simulink model "VehicleFollowing"  (R2020a)
settings: Solver=VariableStepAuto  StartTime=0.0  StopTime=30  RelTol=1e-3
InitFcn:
  | load("bus.mat");
model workspace (MAT data in the model file):
  Acc_command = Simulink.Parameter
  Acc_command.DataType = 'auto'
  Acc_command.Dimensions = [0 0]
  AngIn_command = Simulink.Parameter
  AngIn_command.DataType = 'auto'
  AngIn_command.Dimensions = [0 0]
  Dece_command = Simulink.Parameter
  Dece_command.DataType = 'auto'
  Dece_command.Dimensions = [0 0]
libraries: autolibutils x4, autolibshared x3, simulink x3, drivinglib x2, drivingscenarioandsensors x2, vrlib x2, vehdynlibsteering x1, mpcadaslib x1, robotalgslib x1
(part 1 of 3)
settings Model: PacingRate=1.100000  OrderedModelArguments=off  Creator=shiqihang  LastModifiedBy=shiqihang
settings SolverCC: AlgebraicLoopSolver=LineSearch
settings DebuggingCC: AlgebraicLoopMsg=none

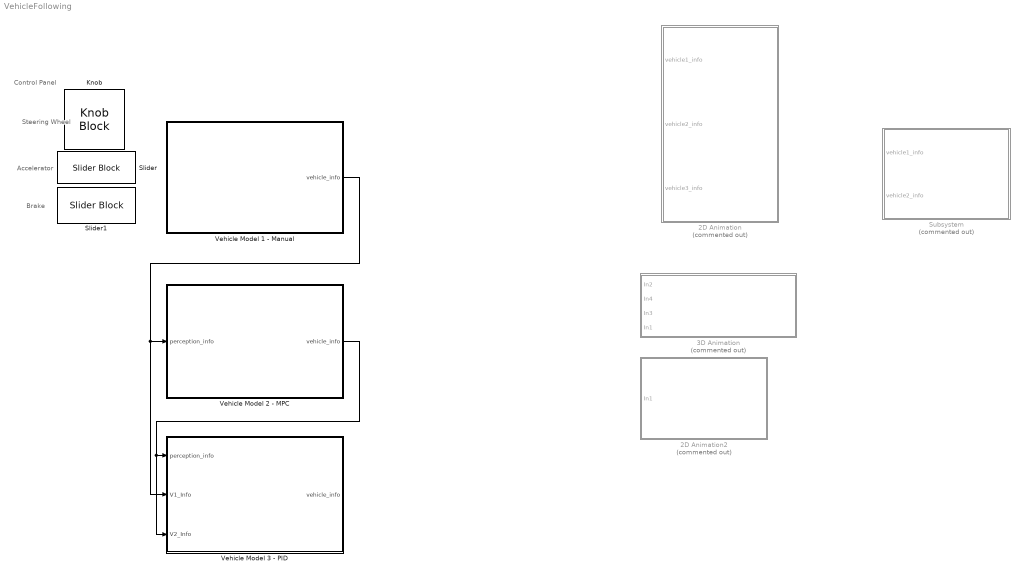
== system VehicleFollowing ==
  note: Steering
      | Wheel
  note: Control Panel
  note: Accelerator
  note: Brake
  2D Animation : Subsystem  Commented=on  TreatAsAtomicUnit=on  SystemSampleTime=0.02
  2D Animation2 : Subsystem  Commented=on
  3D Animation : Subsystem  Commented=on
  Knob : KnobBlock  ScaleMin=-2  ScaleMax=2
  Slider : SliderBlock
  Slider1 : SliderBlock
  Subsystem : Subsystem  Commented=on
  Vehicle Model 1 - Manual : Subsystem  mask{X_init=150, xdot_init=10, Y_init=-2.5, ydot_init=0, AngIn_command=-0.006511027018229143, Acc_command=0.3429878048780488, Dece_command=0}
      mask prompts: X_init "Initial X Position"; xdot_init "Initial Longitudinal Velocity"; Y_init "Initial Y Position"; ydot_init "Initial Lateral Velocity"; AngIn_command "Angle Command"; Acc_command "Acc Command"; Dece_command "Dece Command"
      mask Display: image('$imagefile'); % Use "Edit Image" on toolstrip to change.
  Vehicle Model 2 - MPC : Subsystem  mask{X_init=40, xdot_init=5, Y_init=-2.5, ydot_init=0}
      mask prompts: X_init "Initial X Position"; xdot_init "Initial Longitudinal Velocity"; Y_init "Initial Y Position"; ydot_init "Initial Lateral Velocity"
      mask TypeOptions X_init: Initial Position Z/Value
      mask TypeOptions xdot_init: Initial Speed/Value
      mask Display: image('$imagefile'); % Use "Edit Image" on toolstrip to change.
  Vehicle Model 3 - PID : Subsystem  mask{X_init=0, xdot_init=20, Y_init=-2.5, ydot_init=0}
      mask prompts: X_init "Initial X Position"; xdot_init "Initial Longitudinal Velocity"; Y_init "Initial Y Position"; ydot_init "Initial Lateral Velocity"
      mask TypeOptions X_init: Initial Position Z/Value
      mask TypeOptions xdot_init: Initial Speed/Value
      mask Display: image('C:\Users\qihan\Desktop\Git\Vehicle-following-model-with-3DAnimation\resources\image\vehicle.png'); % Use "Edit Image" on toolstrip to change.
  wires:
  Vehicle Model 1 - Manual/1(vehicle_info) -> Vehicle Model 2 - MPC/1(perception_info), Vehicle Model 3 - PID/2(V1_Info)
  Vehicle Model 2 - MPC/1(vehicle_info) -> Vehicle Model 3 - PID/3(V2_Info), Vehicle Model 3 - PID/1(perception_info)

== system VehicleFollowing/2D Animation ==
  vehicle1_info : Inport
  vehicle2_info : Inport  Port=2
  vehicle3_info : Inport  Port=3
  Bus Selector : BusSelector  OutputSignals=InertFrm.Cg.Disp.X,InertFrm.Cg.Disp.Y,InertFrm.Cg.Ang.psi  OutputAsBus=on
  Bus Selector1 : BusSelector  OutputSignals=X,Y,psi  OutputAsBus=on
  Bus Selector2 : BusSelector  OutputSignals=InertFrm.Cg.Disp.X,InertFrm.Cg.Disp.Y,InertFrm.Cg.Ang.psi  OutputAsBus=on
  MATLAB Function : MATLAB Function  TreatAsAtomicUnit=on
      mask init:
      | close all;
      | figure('units','normalized','outerposition',[0 0 1 1]);
      | grid on
      | axis equal
      | hold on
  wires:
  Bus Selector/1 -> MATLAB Function/1(V1_Pose)
  vehicle1_info/1 -> Bus Selector/1
  vehicle2_info/1 -> Bus Selector1/1
  Bus Selector1/1 -> MATLAB Function/2(V2_Pose)
  vehicle3_info/1 -> Bus Selector2/1
  Bus Selector2/1 -> MATLAB Function/3(V3_Pose)

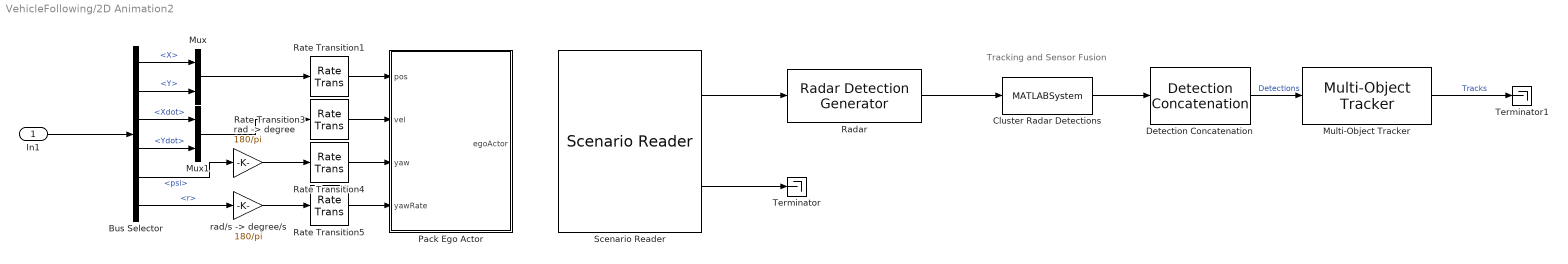
== system VehicleFollowing/2D Animation2 ==
  note: Tracking and Sensor Fusion
  In1 : Inport
  Bus Selector : BusSelector  OutputSignals=InertFrm.Cg.Disp.X,InertFrm.Cg.Disp.Y,InertFrm.Cg.Vel.Xdot,InertFrm.Cg.Vel.Ydot,InertFrm.Cg.Ang.psi,BdyFrm.Cg.AngVel.r
  Cluster Radar Detections : MATLABSystem  System=helperClusterDetections  ClusterSize=5  BusNameSource=Auto  BusName=BusClusterDetections  SimulateUsing=Interpreted execution
      mask Type: helperClusterDetections
      mask Display:
      | disp(['Detection' char(10) 'Clustering']);
      | port_label('input',1,'In');
      | port_label('output',1,'Out');
  Detection Concatenation : drivinglib/Detection Concatenation  NumInputs=1  BusNameSource=Auto  BusName=BusDetectionConcatenation1  SimulateUsing=Interpreted execution
      settings: SourceProductBaseCode=DR
  Multi-Object Tracker : drivinglib/Multi-Object Tracker  TrackerIndex=uint32( 0 )  FilterInitializationFcn=helperInitSimulinkDemoFilter  AssignmentThreshold=50  ConfirmationThreshold=[ 2, 3 ]  DeletionThreshold=[5,5]  MaxNumTracks=20  MaxNumSensors=8  StateParams=struct  TimeInputSource=Auto  HasCostMatrixInput=off  HasDetectableTrackIDsInput=off  BusNameSource=Auto  BusName=BusMultiObjectTracker1  TentativeTracksOutputPort=off  AllTracksOutputPort=off  SimulateUsing=Interpreted execution
      settings: SourceProductBaseCode=DR
  Mux : Mux  Inputs=2
  Mux1 : Mux  Inputs=2
  Pack Ego Actor : MATLAB Function  TreatAsAtomicUnit=on
  Radar : drivingscenarioandsensors/Radar Detection Generator  SensorIndex=1  UpdateInterval=0.1  SensorLocation=[3.7 0]  Height=0.2  Yaw=0  Pitch=0  Roll=0  BusNameSource=Auto  BusName=BusRadarDetectionGenerator  MaxNumDetectionsSource=Property  MaxNumDetections=50  DetectionCoordinates=Ego Cartesian  SimulateUsing=Interpreted execution  AzimuthResolution=4  ElevationResolution=10  RangeResolution=2.5  RangeRateResolution=0.5  AzimuthBiasFraction=0.1  ElevationBiasFraction=0.1  RangeBiasFraction=0.05  RangeRateBiasFraction=0.05  FieldOfView=[20 5]  MaxRange=100  RangeRateLimits=[-100 100]  DetectionProbability=0.9  FalseAlarmRate=1e-06  ReferenceRange=100  ReferenceRCS=0  HasElevation=off  HasRangeRate=on  HasNoise=on  HasFalseAlarms=on  HasOcclusion=on  InitialSeedSource=Repeatable  InitialSeed=0  UsedSeed=0  ActorProfilesSource=MATLAB expression  ActorProfilesParameters=driving.internal.ActorProfilesRadarParameters  ActorProfilesExpression=[struct('ActorID',1,'ClassID',1,'Length',4.7,'Width',1.8,'Height',1.4,'OriginOffset',[-1.35 0 0],'MeshVertices',[3.7 -0.9 1.4;3.7 0.9 1.4;-1 0.9 1.4;-1 -0.9 1.4;3.7 -0.9 0;3.7 0.9 0;-1 0.9 0;-1 -0.9 0],'MeshFaces',[6 2 1;1 5 6;8 4 3;3 7 8;6 7 3;3 2 6;5 1 4;4 8 5;4 1 2;2 3 4;7 6 5;5 8 7],'RCSPattern',[10 10;10 10],'RCSAzimuthAngles',[-180 180],'RCSElevationAngles',[-90 90]); struct('ActorID',2,'ClassID',1,'Length',4.7,'Width',1.8,'Height',1.4,'OriginOffset',[-1.35 0 0],'MeshVertices',[3.7 -0.9 1.4;3.7 0.9 1.4;-1 0.9 1.4;-1 -0.9 1.4;3.7 -0.9 0;3.7 0.9 0;-1 0.9 0;-1 -0.9 0],'MeshFaces',[6 2 1;1 5 6;8 4 3;3 7 8;6 7 3;3 2 6;5 1 4;4 8 5;4 1 2;2 3 4;7 6 5;5 8 7],'RCSPattern',[10 10;10 10],'RCSAzimuthAngles',[-180 180],'RCSElevationAngles',[-90 90]); struct('ActorID',3,'ClassID',1,'Length',4.7,'Width',1.8,'Height',1.4,'OriginOffset',[-1.35 0 0],'MeshVertices',[3.7 -0.9 1.4;3.7 0.9 1.4;-1 0.9 1.4;-1 -0.9 1.4;3.7 -0.9 0;3.7 0.9 0;-1 0.9 0;-1 -0.9 0],'MeshFaces',[6 2 1;1 5 6;8 4 3;3 7 8;6 7 3;3 2 6;5 1 4;4 8 5;4 1 2;2 3 4;7 6 5;5 8 7],'RCSPattern',[10 10;10 10],'RCSAzimuthAngles',[-180 180],'RCSElevationAngles',[-90 90])]
      settings: SourceProductBaseCode=DR
  Rate Transition{1,3..5} (4 alike) : RateTransition  OutPortSampleTime=0.1
  Scenario Reader : drivingscenarioandsensors/Scenario Reader  ScenarioSource=From workspace  ScenarioFileName=C:\Users\qihan\Desktop\Git\Vehicle-following-model-with-3DAnimation\roads.mat  ScenarioVariableName=ans  OutputCoordinateSystem=Vehicle coordinates  EgoVehicleSource=Scenario  OrientVehiclesOnRoad=off  EgoVehicleActorID=1  OutputEgoVehiclePose=off  SampleTime=0.1  LaneBoundaryOutput=Ego vehicle lane boundaries  LaneBoundaryDistance=0:0.5:9.5  LaneBoundaryLocation=Center of lane markings  BusNameSource=Auto  BusName=BusActors  BusName2Source=Auto  BusName2=BusVision1  BusName3Source=Auto  BusName3=BusEgoActor  ShowCoordinateLabels=on  SimulateUsing=Interpreted execution
  Terminator : Terminator
  Terminator1 : Terminator
  "rad -> degree" : Gain  Gain=180/pi
  "rad/s -> degree/s" : Gain  Gain=180/pi
  wires:
  Rate Transition1/1 -> Pack Ego Actor/1(pos)
  Mux/1 -> Rate Transition1/1
  Multi-Object Tracker/1 -> Terminator1/1  "Tracks"
  "rad -> degree"/1 -> Rate Transition4/1
  Bus Selector/1 -> Mux/1  "<X>"
  Rate Transition5/1 -> Pack Ego Actor/4(yawRate)
  Mux1/1 -> Rate Transition3/1
  "rad/s -> degree/s"/1 -> Rate Transition5/1
  Bus Selector/5 -> "rad -> degree"/1  "<psi>"
  Bus Selector/4 -> Mux1/2  "<Ydot>"
  Scenario Reader/1 -> Radar/1
  Bus Selector/3 -> Mux1/1  "<Xdot>"
  Bus Selector/2 -> Mux/2  "<Y>"
  Rate Transition3/1 -> Pack Ego Actor/2(vel)
  Bus Selector/6 -> "rad/s -> degree/s"/1  "<r>"
  Detection Concatenation/1 -> Multi-Object Tracker/1  "Detections"
  Scenario Reader/2 -> Terminator/1
  Radar/1 -> Cluster Radar Detections/1
  Cluster Radar Detections/1 -> Detection Concatenation/1
  Rate Transition4/1 -> Pack Ego Actor/3(yaw)
  In1/1 -> Bus Selector/1

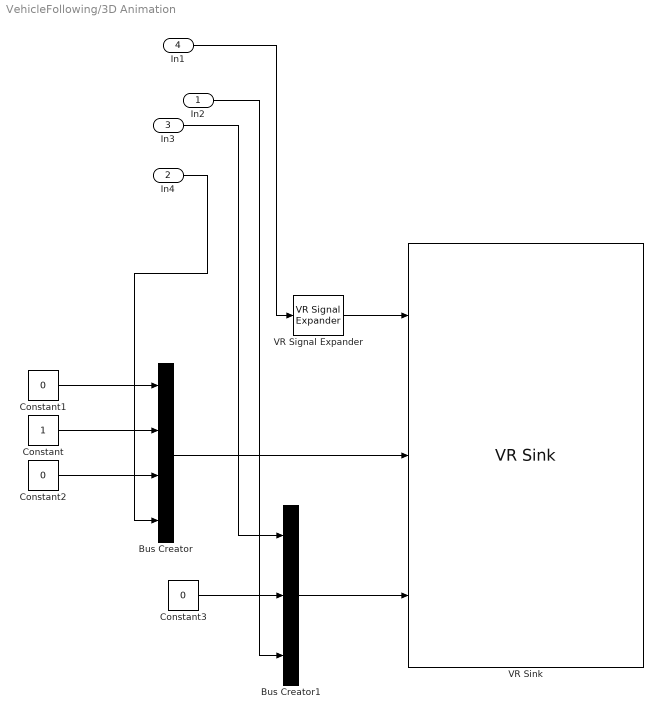
== system VehicleFollowing/3D Animation ==
  In2 : Inport
  In4 : Inport  Port=2
  In3 : Inport  Port=3
  In1 : Inport  Port=4
  Bus Creator : BusCreator  Inputs=4
  Bus Creator1 : BusCreator  Inputs=3
  Constant : Constant
  Constant1 : Constant  Value=0
  Constant2 : Constant  Value=0
  Constant3 : Constant  Value=0
  VR Signal Expander : vrlib/VR Signal Expander  outwidth=3  outidx=[3]
  VR Sink : vrlib/VR Sink  InstantiateOnLoad=on  SampleTime=0.02  ViewEnable=on  RemoteChange=off  RemoteView=off  FieldsWritten=Car_Red.translation.3.1.1.double#Car_Blue.rotation.4.1.1.double#Car_Blue.translation.3.1.1.double  WorldFileName=PlatoonWorld.WRL  AutoView=off  VideoDimensions=[]  AllowVariableSize=off
  wires:
  Constant/1 -> Bus Creator/2
  Constant1/1 -> Bus Creator/1
  Bus Creator1/1 -> VR Sink/3
  In2/1 -> Bus Creator1/3
  Bus Creator/1 -> VR Sink/2
  In4/1 -> Bus Creator/4
  In1/1 -> VR Signal Expander/1
  Constant3/1 -> Bus Creator1/2
  Constant2/1 -> Bus Creator/3
  VR Signal Expander/1 -> VR Sink/1
  In3/1 -> Bus Creator1/1

== system VehicleFollowing/Subsystem ==
  vehicle1_info : Inport
  vehicle2_info : Inport  Port=2
  Bus Selector : BusSelector  OutputSignals=InertFrm.Cg.Disp.X,InertFrm.Cg.Disp.Y,InertFrm.Cg.Ang.psi  OutputAsBus=on
  Bus Selector1 : BusSelector  OutputSignals=X,Y,psi  OutputAsBus=on
  Collision Detection : MATLABSystem  System=collision_detection  v1_frame=[ 4, 2 ]  v2_frame=[ 4, 2 ]  SimulateUsing=Interpreted execution
      mask Type: collision_detection
      mask Display:
      | disp('collision_detection');
      | port_label('input',1,'v1_pos');
      | port_label('input',2,'v2_pos');
      | port_label('output',1,'collision_flag');
  Stop Simulation : Stop
  wires:
  Collision Detection/1 -> Stop Simulation/1
  vehicle1_info/1 -> Bus Selector/1
  Bus Selector1/1 -> Collision Detection/2
  Bus Selector/1 -> Collision Detection/1
  vehicle2_info/1 -> Bus Selector1/1

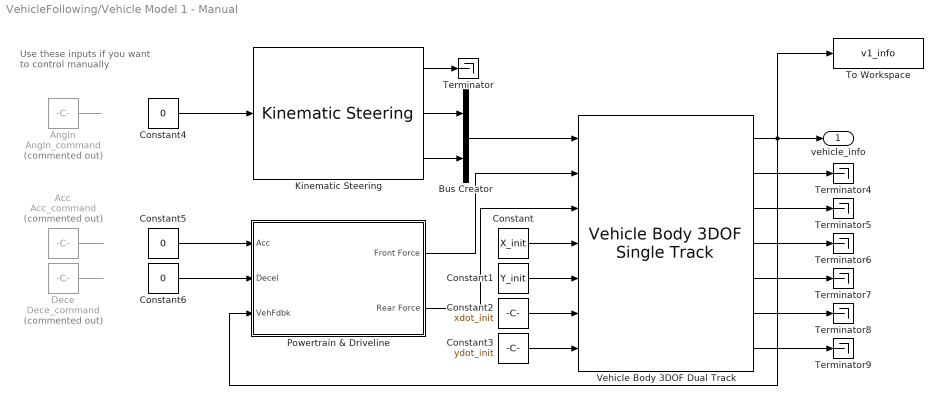
== system VehicleFollowing/Vehicle Model 1 - Manual ==
  note: Use these inputs if
      | you want to control
      | manually
  Acc : Constant  Commented=on  Value=Acc_command
  AngIn : Constant  Commented=on  Value=AngIn_command
  Bus Creator : BusCreator  Inputs=2
  Constant : Constant  Value=X_init
  Constant1 : Constant  Value=Y_init
  Constant2 : Constant  Value=xdot_init
  Constant3 : Constant  Value=ydot_init
  Constant4 : Constant  Value=0
  Constant5 : Constant  Value=0
  Constant6 : Constant  Value=0
  Dece : Constant  Commented=on  Value=Dece_command
  Kinematic Steering : vehdynlibsteering/Kinematic Steering  StrgType=Rack and pinion  StrgRatioType=Constant  Loc=Front  NrmlFctr=0.01  TrckWdth=1  WhlBase=1.524  Db=0  StrgRng=1.25*pi  StrgAngBpts="[-6.2832   -5.0265   -3.7699   -2.5133   -1.2566         0    1.2566    2.5133    3.7699    5.0265    6.2832]"  StrgRatioTbl=|  StrgRatio=100  StrgArmLngth=0.1  RckCsLngth=0.5  TieRodLngth=0.248  D=0.2  PnnRadius=0.0057  PnnRadiusTbl="[0.0055    0.0055    0.0056    0.0057    0.0058    0.0057    0.0057    0.0057    0.0056    0.0055    0.0055]"  RodLngth=0.1  ParaArmLngth=0.9  aMode=2
      | [13.5000   13.3750   13.2500   13.1250   13.0000   13.0000   13.0000   13.1250   13.2500   13.3750   13.5000
      | ]
  Powertrain & Driveline : Subsystem
      mask Display: image('vdbslibpt.png');
  Terminator{,4..9} (7 alike) : Terminator
  To Workspace : ToWorkspace  VariableName=v1_info  SaveFormat=Timeseries  SampleTime=0.1
  Vehicle Body 3DOF Dual Track : autolibshared/Vehicle Body 3DOF Single Track  trackMode=Dual  inputMode=External longitudinal forces  frontSteerMode=on  rearSteerMode=off  windMode=off  muMode=off  extFMode=off  extMMode=off  extXo=on  extpsio=off  extxdoto=on  extro=off  extYo=on  extTamb=off  extydoto=on  aMode=2  NF=2  NR=2  m=2000  a=1.4  b=1.6  h=0.35  X_o=0  xdot_o=0  CalphaMode=off  sigmaMode=on  d=0  w=[1.4,1.4]  Cy_f=12e3  Cy_r=11e3  sigma_f=.1  sigma_r=.1  alpha_f_brk=[-.1 .1]  Cy_f_data=[-9e3 9e3]  alpha_r_brk=[-.1 .1]  Cy_r_data=[-9e3 9e3]  Y_o=0  ydot_o=0  Izz=4000  psi_o=0  r_o=0  Af=2  Cd=.3  Cl=.1  Cpm=.1  beta_w=[0:0.01:0.3]  Cs=[0:0.03:0.9]  Cym=[0:0.01:0.3]  Pabs=101325  Tair=273  g=9.81  mu=1  xdot_tol=.01  Fznom=5000  Fxtire_sat=7e4  Fytire_sat=7e4  longOff=0  latOff=0  vertOff=0  wrapAng=off
      settings: SourceProductBaseCode=PW,MT,VE,VP
  vehicle_info : Outport
  wires:
  Dece/1 -> ?
  AngIn/1 -> ?
  Kinematic Steering/3 -> Bus Creator/2
  Vehicle Body 3DOF Dual Track/4 -> Terminator6/1
  Acc/1 -> ?
  Vehicle Body 3DOF Dual Track/2 -> Terminator4/1
  Vehicle Body 3DOF Dual Track/6 -> Terminator8/1
  Powertrain & Driveline/2(Rear Force) -> Vehicle Body 3DOF Dual Track/3
  Vehicle Body 3DOF Dual Track/1 -> To Workspace/1, Powertrain & Driveline/3(VehFdbk), vehicle_info/1
  Vehicle Body 3DOF Dual Track/5 -> Terminator7/1
  Powertrain & Driveline/1(Front Force) -> Vehicle Body 3DOF Dual Track/2
  Kinematic Steering/1 -> Terminator/1
  Vehicle Body 3DOF Dual Track/3 -> Terminator5/1
  Bus Creator/1 -> Vehicle Body 3DOF Dual Track/1
  Vehicle Body 3DOF Dual Track/7 -> Terminator9/1
  Kinematic Steering/2 -> Bus Creator/1
  Constant3/1 -> Vehicle Body 3DOF Dual Track/7
  Constant2/1 -> Vehicle Body 3DOF Dual Track/6
  Constant1/1 -> Vehicle Body 3DOF Dual Track/5
  Constant/1 -> Vehicle Body 3DOF Dual Track/4
  Constant4/1 -> Kinematic Steering/1
  Constant6/1 -> Powertrain & Driveline/2(Decel)
  Constant5/1 -> Powertrain & Driveline/1(Acc)

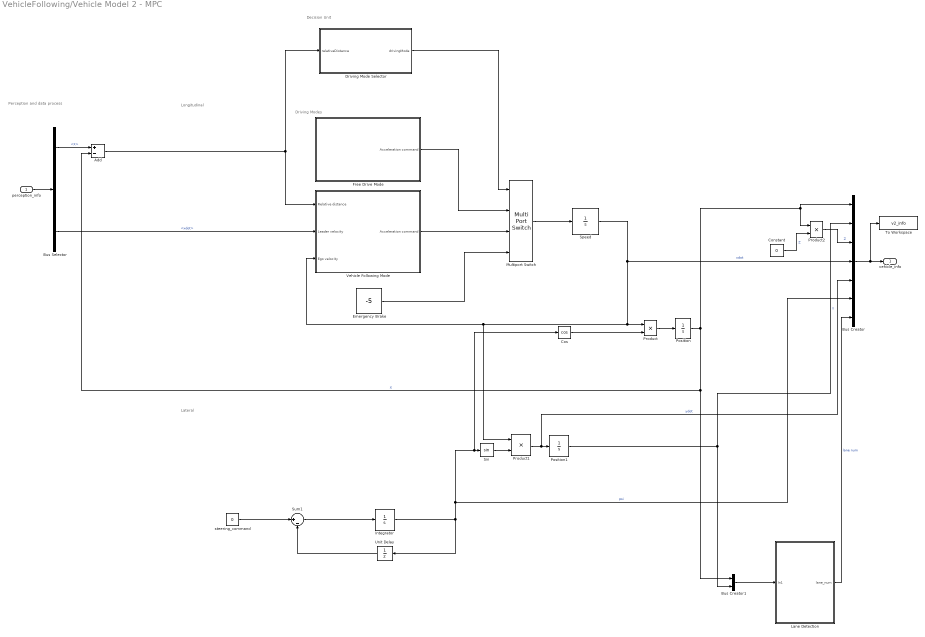
== system VehicleFollowing/Vehicle Model 2 - MPC ==
  note: Perception and data process
  note: Lateral
  note: Longitudinal
  note: Driving Modes
  note: Decision Unit
  perception_info : Inport
  Add : Sum  Inputs=+-
  Bus Creator : BusCreator  Inputs=7
  Bus Creator1 : BusCreator  Inputs=2
  Bus Selector : BusSelector  OutputSignals=InertFrm.Cg.Disp.X,InertFrm.Cg.Disp.Y,BdyFrm.Cg.Vel.xdot
  Constant : Constant  Value=0
  Cos : Trigonometry  Operator=cos
  Driving Mode Selector : Stateflow chart  TreatAsAtomicUnit=on
  Emergency Brake : Constant  Value=-5
  Free Drive Mode : Subsystem
  Integrator : Integrator
  Lane Detection : Subsystem
  Multiport Switch : MultiPortSwitch
  Position : Integrator  InitialCondition=X_init
  Position1 : Integrator  InitialCondition=Y_init
  Product : Product
  Product1 : Product
  Product2 : Product
  Sin : Trigonometry
  Speed : Integrator  InitialCondition=xdot_init  LimitOutput=on  LowerSaturationLimit=0
  Sum1 : Sum  Inputs=|+-
  To Workspace : ToWorkspace  VariableName=v2_info  SaveFormat=Timeseries  SampleTime=-1
  Unit Delay : UnitDelay  SampleTime=-1  HasFrameUpgradeWarning=on
  Vehicle Following Mode : Subsystem
  steering_command : Constant  Value=0
  vehicle_info : Outport
  wires:
  Driving Mode Selector/1(drivingMode) -> Multiport Switch/1
  Emergency Brake/1 -> Multiport Switch/4
  Free Drive Mode/1(Acceleration command) -> Multiport Switch/2
  Multiport Switch/1 -> Speed/1
  Vehicle Following Mode/1(Acceleration command) -> Multiport Switch/3
  Bus Selector/3 -> Vehicle Following Mode/2(Leader velocity)  "<xdot>"
  Add/1 -> Vehicle Following Mode/1(Relative distance), Driving Mode Selector/1(relativeDistance)
  Position1/1 -> Bus Creator1/2, Bus Creator/2  "Y"
  Product1/1 -> Bus Creator/5, Position1/1  "ydot"
  Sin/1 -> Product1/2
  Product/1 -> Position/1
  Cos/1 -> Product/2
  Unit Delay/1 -> Sum1/2
  Integrator/1 -> Bus Creator/6, Cos/1, Sin/1, Unit Delay/1  "psi"
  Sum1/1 -> Integrator/1
  steering_command/1 -> Sum1/1
  Speed/1 -> Product1/1, Vehicle Following Mode/3(Ego velocity), Product/1, Bus Creator/4  "xdot"
  Position/1 -> Product2/1, Bus Creator/1, Bus Creator1/1, Add/2  "X"
  perception_info/1 -> Bus Selector/1
  Bus Selector/1 -> Add/1  "<X>"
  Bus Creator/1 -> To Workspace/1, vehicle_info/1
  Product2/1 -> Bus Creator/3  "Z"
  Constant/1 -> Product2/2  "Z"
  Bus Creator1/1 -> Lane Detection/1(In1)
  Lane Detection/1(lane_num) -> Bus Creator/7  "lane num"

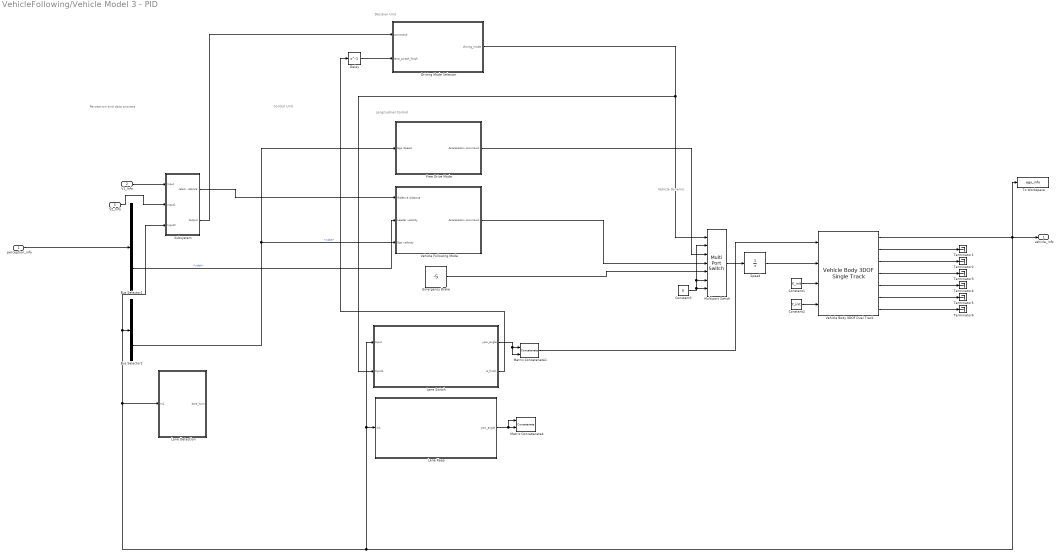
== system VehicleFollowing/Vehicle Model 3 - PID ==
  note: Vehicle Dynamic
  note: Decision Unit
  note: Control Unit
  note: Perception and data process
  note: Longitudinal Control
  perception_info : Inport
  V1_Info : Inport  Port=2
  V2_Info : Inport  Port=3
  Bus Selector1 : BusSelector  OutputSignals=X,xdot
  Bus Selector2 : BusSelector  OutputSignals=InertFrm.Cg.Disp.X,BdyFrm.Cg.Vel.xdot
  Constant1 : Constant  Value=X_init
  Constant2 : Constant  Value=Y_init
  Constant3 : Constant  Value=0
  Delay : Delay  DelayLength=1
  Driving Mode Selector : Stateflow chart  TreatAsAtomicUnit=on
  Emergency Brake : Constant  Value=-5
  Free Drive Mode : Subsystem
  Lane Detection : Subsystem
  Lane Keep : Subsystem
  Lane Switch : Subsystem
  Matrix Concatenate1 : Concatenate  Mode=Multidimensional array  ConcatenateDimension=2
  Matrix Concatenate4 : Concatenate  Mode=Multidimensional array  ConcatenateDimension=2
  Multiport Switch : MultiPortSwitch  DataPortOrder=Zero-based contiguous  Inputs=6  zeroidx=on
  Speed : Integrator  InitialCondition=xdot_init  LimitOutput=on  LowerSaturationLimit=0
  Subsystem : Subsystem
  Terminator{1..6} (6 alike) : Terminator
  To Workspace : ToWorkspace  VariableName=ego_info  SaveFormat=Timeseries  SampleTime=0.1
  Vehicle Body 3DOF Dual Track : autolibshared/Vehicle Body 3DOF Single Track  trackMode=Dual  inputMode=External longitudinal velocity  frontSteerMode=on  rearSteerMode=off  windMode=off  muMode=off  extFMode=off  extMMode=off  extXo=on  extpsio=off  extxdoto=off  extro=off  extYo=on  extTamb=off  extydoto=off  aMode=2  NF=2  NR=2  m=2000  a=1.4  b=1.6  h=0.35  X_o=0  xdot_o=0  CalphaMode=off  sigmaMode=on  d=0  w=[1.4,1.4]  Cy_f=12e3  Cy_r=11e3  sigma_f=.1  sigma_r=.1  alpha_f_brk=[-.1 .1]  Cy_f_data=[-9e3 9e3]  alpha_r_brk=[-.1 .1]  Cy_r_data=[-9e3 9e3]  Y_o=0  ydot_o=0  Izz=4000  psi_o=0  r_o=0  Af=2  Cd=.3  Cl=.1  Cpm=.1  beta_w=[0:0.01:0.3]  Cs=[0:0.03:0.9]  Cym=[0:0.01:0.3]  Pabs=101325  Tair=273  g=9.81  mu=1  xdot_tol=.01  Fznom=5000  Fxtire_sat=7e4  Fytire_sat=7e4  longOff=0  latOff=0  vertOff=0  wrapAng=off
      settings: SourceProductBaseCode=PW,MT,VE,VP
  Vehicle Following Mode : Subsystem
  vehicle_info : Outport
  wires:
  Speed/1 -> Vehicle Body 3DOF Dual Track/2
  Bus Selector1/2 -> Vehicle Following Mode/2(Leader velocity)  "<xdot>"
  Vehicle Following Mode/1(Acceleration command) -> Multiport Switch/4
  Multiport Switch/1 -> Speed/1
  Free Drive Mode/1(Acceleration command) -> Multiport Switch/3
  Emergency Brake/1 -> Multiport Switch/5
  Vehicle Body 3DOF Dual Track/1 -> Lane Switch/1(Input), Lane Keep/1(In1), Lane Detection/1(In1), Subsystem/3(Input2), Bus Selector2/1, To Workspace/1, vehicle_info/1
  Vehicle Body 3DOF Dual Track/2 -> Terminator1/1
  Vehicle Body 3DOF Dual Track/3 -> Terminator2/1
  Vehicle Body 3DOF Dual Track/4 -> Terminator3/1
  Vehicle Body 3DOF Dual Track/5 -> Terminator4/1
  Vehicle Body 3DOF Dual Track/6 -> Terminator5/1
  Vehicle Body 3DOF Dual Track/7 -> Terminator6/1
  Constant1/1 -> Vehicle Body 3DOF Dual Track/3
  Constant2/1 -> Vehicle Body 3DOF Dual Track/4
  Constant3/1 -> Multiport Switch/2, Multiport Switch/6, Multiport Switch/7
  Driving Mode Selector/1(driving_mode) -> Lane Switch/2(Input1), Multiport Switch/1
  perception_info/1 -> Bus Selector1/1
  Bus Selector2/2 -> Vehicle Following Mode/3(Ego velocity), Free Drive Mode/1(Ego Speed)  "<xdot>"
  Lane Keep/1(yaw_angle) -> Matrix Concatenate4/2, Matrix Concatenate4/1
  Lane Switch/1(yaw_angle) -> Matrix Concatenate1/2, Matrix Concatenate1/1
  Matrix Concatenate1/1 -> Vehicle Body 3DOF Dual Track/1
  Subsystem/1(relative_distance) -> Vehicle Following Mode/1(Relative distance)
  Lane Switch/2(is_finish) -> Delay/1
  Delay/1 -> Driving Mode Selector/2(lane_switch_finish)
  V1_Info/1 -> Subsystem/1(Input)
  V2_Info/1 -> Subsystem/2(Input1)
  Subsystem/2(Output) -> Driving Mode Selector/1(command)

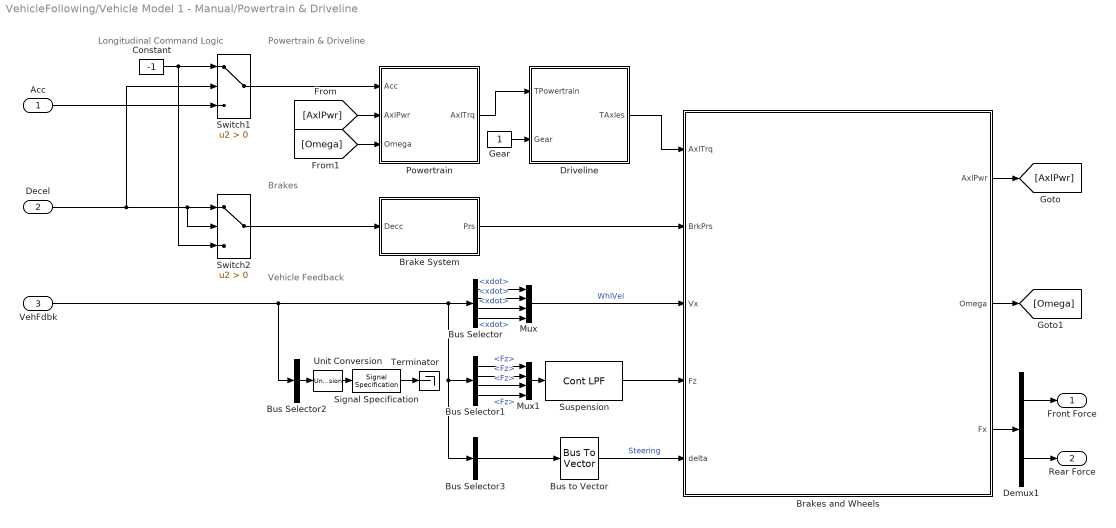
== system VehicleFollowing/Vehicle Model 1 - Manual/Powertrain & Driveline ==
  note: Longitudinal Command Logic
  note: Brakes
  note: Powertrain & Driveline
  note: Vehicle Feedback
  Acc : Inport
  Decel : Inport  Port=2
  VehFdbk : Inport  Port=3
  Brake System : Subsystem
  Brakes and Wheels : Subsystem  TreatAsAtomicUnit=on
      mask Display: image('vdbslibwhls.png');
  Bus Selector : BusSelector  OutputSignals=BdyFrm.FrntAxl.Lft.Vel.xdot,BdyFrm.FrntAxl.Rght.Vel.xdot,BdyFrm.RearAxl.Lft.Vel.xdot,BdyFrm.RearAxl.Rght.Vel.xdot
  Bus Selector1 : BusSelector  OutputSignals=BdyFrm.Forces.FrntAxl.Lft.Fz,BdyFrm.Forces.FrntAxl.Rght.Fz,BdyFrm.Forces.RearAxl.Lft.Fz,BdyFrm.Forces.RearAxl.Rght.Fz
  Bus Selector2 : BusSelector  OutputSignals=BdyFrm.Cg.Vel.xdot  OutputAsBus=on
  Bus Selector3 : BusSelector  OutputSignals=BdyFrm.FrntAxl.Steer.WhlAngFL,BdyFrm.FrntAxl.Steer.WhlAngFR,BdyFrm.RearAxl.Steer.WhlAngRL,BdyFrm.RearAxl.Steer.WhlAngRR  OutputAsBus=on
  Bus to Vector : BusToVector
  Constant : Constant  Value=-1
  Demux1 : Demux  Outputs=[2 2]
  Driveline : Subsystem  Variant=on  VariantControlMode=Label  VariantControl=Variant1  LabelModeActiveChoice=0
  Gear : Constant
  Mux : Mux
  Mux1 : Mux
  Powertrain : Subsystem
  Signal Specification : SignalSpecification  Unit=km/hr
  Suspension : autolibutils/Cont LPF  wc=10*pi*2  aMode=2
      settings: SourceProductBaseCode=PW,MT,VE,VP
  Switch1 : Switch  Criteria=u2 > Threshold
  Switch2 : Switch  Criteria=u2 > Threshold
  Terminator : Terminator
  Unit Conversion : UnitConversion
  Front Force : Outport  VectorParamsAs1DForOutWhenUnconnected=off
  Rear Force : Outport  Port=2  VectorParamsAs1DForOutWhenUnconnected=off
  wires:
  Decel/1 -> Switch1/2, Switch2/2, Switch2/1
  Acc/1 -> Switch1/3
  Constant/1 -> Switch2/3, Switch1/1
  Mux/1 -> Brakes and Wheels/3(Vx)  "WhlVel"
  VehFdbk/1 -> Bus Selector2/1, Bus Selector3/1, Bus Selector1/1, Bus Selector/1
  Demux1/1 -> Front Force/1
  Demux1/2 -> Rear Force/1
  Driveline/1(TAxles) -> Brakes and Wheels/1(AxlTrq)
  Brakes and Wheels/1(AxlPwr) -> [AxlPwr]
  Brakes and Wheels/3(Fx) -> Demux1/1
  Bus Selector3/1 -> Bus to Vector/1
  Bus to Vector/1 -> Brakes and Wheels/5(delta)  "Steering"
  Mux1/1 -> Suspension/1
  Suspension/1 -> Brakes and Wheels/4(Fz)
  Bus Selector/1 -> Mux/1  "<xdot>"
  Bus Selector/2 -> Mux/2  "<xdot>"
  Bus Selector/3 -> Mux/3  "<xdot>"
  Bus Selector/4 -> Mux/4  "<xdot>"
  Bus Selector1/1 -> Mux1/1  "<Fz>"
  Bus Selector1/2 -> Mux1/2  "<Fz>"
  Bus Selector1/3 -> Mux1/3  "<Fz>"
  Bus Selector1/4 -> Mux1/4  "<Fz>"
  Switch1/1 -> Powertrain/1(Acc)
  Powertrain/1(AxlTrq) -> Driveline/1(TPowertrain)
  Brakes and Wheels/2(Omega) -> [Omega]
  [AxlPwr] -> Powertrain/2(AxlPwr)
  [Omega] -> Powertrain/3(Omega)
  Switch2/1 -> Brake System/1(Decc)
  Brake System/1(Prs) -> Brakes and Wheels/2(BrkPrs)
  Bus Selector2/1 -> Unit Conversion/1
  Unit Conversion/1 -> Signal Specification/1
  Signal Specification/1 -> Terminator/1
  Gear/1 -> Driveline/2(Gear)

== system VehicleFollowing/Vehicle Model 2 - MPC/Free Drive Mode ==
  Acc Command : Saturate  UpperLimit=2  LowerLimit=-3
  Acc Dynamics : TransferFcn  Denominator=[0.5 1]
  Constant : Constant  Value=xdot_init
  Sum13 : Sum  Inputs=|+-
  Acceleration command : Outport
  wires:
  Acc Command/1 -> Acc Dynamics/1
  Constant/1 -> Sum13/1
  Acc Dynamics/1 -> Sum13/2, Acceleration command/1
  Sum13/1 -> Acc Command/1

== system VehicleFollowing/Vehicle Model 2 - MPC/Lane Detection ==
  In1 : Inport
  Bus Selector : BusSelector  OutputSignals=X,Y
  MATLAB System : MATLABSystem  System=lane_localization  SimulateUsing=Code generation
      mask Type: lane_localization
      mask Display:
      | disp('lane_localization');
      | port_label('input',1,'X');
      | port_label('input',2,'Y');
      | port_label('output',1,'lane_property');
  lane_num : Outport
  wires:
  Bus Selector/2 -> MATLAB System/2  "<Y>"
  Bus Selector/1 -> MATLAB System/1  "<X>"
  MATLAB System/1 -> lane_num/1
  In1/1 -> Bus Selector/1

== system VehicleFollowing/Vehicle Model 2 - MPC/Vehicle Following Mode ==
  Relative distance : Inport
  Leader velocity : Inport  Port=2
  Ego velocity : Inport  Port=3
  Acc Dynamics : TransferFcn  Denominator=[0.5 1]
  Adaptive Cruise Control System : mpcadaslib/Adaptive Cruise Control System  EgoModel=tf(1,[0.5,1,0])  InitialEgoVelocity=xdot_init  DefaultSpacing=10  MaxVelocity=50  MinAcceleration=-3  amin_ext=off  MaxAcceleration=2  amax_ext=off  Ts=0.5  PredictionHorizon=200  ControllerBehavior=0.590  suboptimal=off  maxiter=100  datatypeopt=double  optmode=off  trackmode=off
  Headway Time : Constant  Value=2
  Reference Velocity : Constant  Value=30
  Sum13 : Sum  Inputs=|+-
  Acceleration command : Outport
  wires:
  Acc Dynamics/1 -> Acceleration command/1
  Adaptive Cruise Control System/1 -> Acc Dynamics/1
  Relative distance/1 -> Adaptive Cruise Control System/4
  Sum13/1 -> Adaptive Cruise Control System/5
  Ego velocity/1 -> Sum13/2, Adaptive Cruise Control System/3
  Reference Velocity/1 -> Adaptive Cruise Control System/1
  Headway Time/1 -> Adaptive Cruise Control System/2
  Leader velocity/1 -> Sum13/1

== system VehicleFollowing/Vehicle Model 3 - PID/Free Drive Mode ==
  Ego Speed : Inport
  Acc Command : Saturate  UpperLimit=2  LowerLimit=-3
  Acc Dynamics : TransferFcn  Denominator=[0.5 1]
  Constant : Constant  Value=xdot_init
  Sum13 : Sum  Inputs=|+-
  Acceleration command : Outport
  wires:
  Sum13/1 -> Acc Command/1
  Acc Dynamics/1 -> Acceleration command/1
  Constant/1 -> Sum13/1
  Acc Command/1 -> Acc Dynamics/1
  Ego Speed/1 -> Sum13/2

== system VehicleFollowing/Vehicle Model 3 - PID/Lane Detection ==
  In1 : Inport
  Bus Selector : BusSelector  OutputSignals=InertFrm.Cg.Disp.X,InertFrm.Cg.Disp.Y
  MATLAB System : MATLABSystem  System=lane_localization  SimulateUsing=Code generation
      mask Type: lane_localization
      mask Display:
      | disp('lane_localization');
      | port_label('input',1,'X');
      | port_label('input',2,'Y');
      | port_label('output',1,'lane_property');
  lane_num : Outport
  wires:
  Bus Selector/2 -> MATLAB System/2  "<Y>"
  Bus Selector/1 -> MATLAB System/1  "<X>"
  MATLAB System/1 -> lane_num/1
  In1/1 -> Bus Selector/1

== system VehicleFollowing/Vehicle Model 3 - PID/Lane Keep ==
  In1 : Inport
  Bus Selector : BusSelector  OutputSignals=InertFrm.Cg.Disp.X,InertFrm.Cg.Disp.Y,InertFrm.Cg.Ang.psi
  MATLAB System1 : MATLABSystem  System=lane_keeping_waypoints_generator  SimulateUsing=Code generation
      mask Type: lane_keeping_waypoints_generator
      mask Display:
      | disp('lane_keeping_waypoints_generator');
      | port_label('input',1,'pos');
      | port_label('output',1,'way_point');
  Mux : Mux  Inputs=3
  Pure Pursuit : robotalgslib/Pure Pursuit  DesiredLinearVelocity=0.1  MaxAngularVelocity=1.0  LookaheadDistance=4  TargetDirPort=on  SimulateUsing=Code generation
  Terminator : Terminator
  Terminator1 : Terminator
  Wheel Steering Angle Formulation : Subsystem  mask{L=4, ld=4}
      mask prompts: L "Bicycle length"; ld "Lookahead distance"
      mask TypeOptions L: Bicycle length/Value
      mask TypeOptions ld: Lookahead distance/Value
      mask Display:
      | image("resources/image/GeometryMask.png")
      | port_label('input', 1, 'alpha')
      | port_label('output', 1, 'delta')
  yaw_angle : Outport
  wires:
  In1/1 -> Bus Selector/1
  Pure Pursuit/3 -> Wheel Steering Angle Formulation/1(alpha)
  Bus Selector/1 -> MATLAB System1/1, Mux/1  "<X>"
  Mux/1 -> Pure Pursuit/1
  MATLAB System1/1 -> Pure Pursuit/2
  Bus Selector/3 -> Mux/3  "<psi>"
  Bus Selector/2 -> Mux/2  "<Y>"
  Wheel Steering Angle Formulation/1(yaw_angle) -> yaw_angle/1
  Pure Pursuit/2 -> Terminator1/1
  Pure Pursuit/1 -> Terminator/1

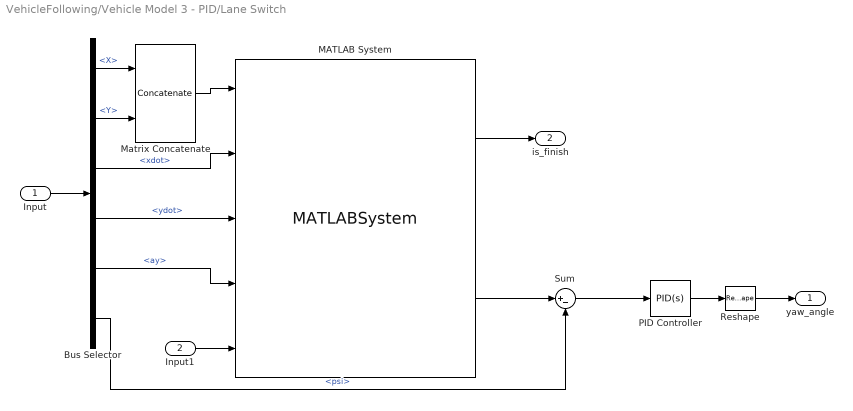
== system VehicleFollowing/Vehicle Model 3 - PID/Lane Switch ==
  Input : Inport
  Input1 : Inport  Port=2
  Bus Selector : BusSelector  OutputSignals=InertFrm.Cg.Disp.X,InertFrm.Cg.Disp.Y,BdyFrm.Cg.Vel.xdot,BdyFrm.Cg.Vel.ydot,BdyFrm.Cg.Acc.ay,InertFrm.Cg.Ang.psi
  MATLAB System : MATLABSystem  System=trajectory_generator  SimulateUsing=Interpreted execution
      mask Type: trajectory_generator
      mask Display:
      | disp('trajectory_generator');
      | port_label('input',1,'current_point');
      | port_label('input',2,'v_x');
      | port_label('input',3,'v_y');
      | port_label('input',4,'a_y');
      | port_label('input',5,'drivingMode');
      | port_label('output',1,'is_finish');
      | port_label('output',2,'yaw_angle');
  Matrix Concatenate : Concatenate  Mode=Multidimensional array  ConcatenateDimension=2
  PID Controller : simulink/Continuous/PID Controller  Controller=PID  Form=Parallel  TimeDomain=Continuous-time  UseExternalTs=off  SampleTime=-1  IntegratorMethod=Forward Euler  FilterMethod=Forward Euler  ControllerParametersSource=internal  P=2  I=1  D=0  UseFilter=on  N=100  TunerSelectOption=Transfer Function Based (PID Tuner App)  InitialConditionSource=internal  InitialConditionForIntegrator=0  InitialConditionForFilter=0  DifferentiatorICPrevScaledInput=0  ExternalReset=none  TrackingMode=off  Kt=1  LimitOutput=off  UpperSaturationLimit=inf  LowerSaturationLimit=-inf  LinearizeAsGain=on  AntiWindupMode=none  Kb=1  POutMin=[]  POutMax=[]  IOutMin=[]  IOutMax=[]  DOutMin=[]  DOutMax=[]  NOutMin=[]  NOutMax=[]  SumOutMin=[]  SumOutMax=[]  SaturationOutMin=[]  SaturationOutMax=[]  PParamMin=[]  PParamMax=[]  IParamMin=[]  IParamMax=[]  DParamMin=[]  DParamMax=[]  NParamMin=[]  NParamMax=[]  KbParamMin=[]  KbParamMax=[]  KtParamMin=[]  KtParamMax=[]  KbOutMin=[]  KbOutMax=[]  KtOutMin=[]  KtOutMax=[]  IntegratorOutMin=[]  IntegratorOutMax=[]  FilterOutMin=[]  FilterOutMax=[]  SumI1OutMin=[]  SumI1OutMax=[]  SumI2OutMin=[]  SumI2OutMax=[]  SumI3OutMin=[]  SumI3OutMax=[]  SumI4OutMin=[]  SumI4OutMax=[]  SumDOutMin=[]  SumDOutMax=[]  DifferentiatorOutMin=[]  DifferentiatorOutMax=[]  FilterDiffOutCoefMin=[]  FilterDiffOutCoefMax=[]  ReciprocalOutMin=[]  ReciprocalOutMax=[]  SumDenOutMin=[]  SumDenOutMax=[]  SumNumOutMin=[]  SumNumOutMax=[]  DivideOutMin=[]  DivideOutMax=[]  UdiffTsProdOutMin=[]  UdiffTsProdOutMax=[]  NTsProdOutMin=[]  NTsProdOutMax=[]  UintegralTsProdOutMin=[]  UintegralTsProdOutMax=[]  UngainTsProdOutMin=[]  UngainTsProdOutMax=[]  IntegratorContinuousStateAttributes=''  IntegratorStateMustResolveToSignalObject=off  IntegratorRTWStateStorageClass=Auto  FilterContinuousStateAttributes=''  FilterStateMustResolveToSignalObject=off  FilterRTWStateStorageClass=Auto  ParallelPVariant=InternalParameters  IdealPVariant=Disabled  IVariant=InternalParameters  DVariant=InternalParameters  IntegratorVariant=Continuous  SatVariant=Disabled  AWVariant=Passthrough  PCopyVariant=Disabled  TRVariant=Disabled  FdbkBlocksVariant=Forward  IdealPFdbkVariant=Disabled  SatFdbkVariant=Disabled  DerivativeFilterVariant=ContFilter  NVariant=InternalParameters  NCopyVariant=Disabled  FilterICVariant=InternalICsFilter  IntegratorICVariant=InternalICs  ExternalResetVariant=Disabled  TRSumVariant=Passthrough  SumFdbkVariant=Disabled  SumVariant=Sum_PID  TsampFilterVariant=InternalTs  TsampNgainVariant=Passthrough  TsampIntegralVariant=Passthrough
  Reshape : Reshape  OutputDimensionality=Customize
  Sum : Sum  Inputs=|+-
  yaw_angle : Outport
  is_finish : Outport  Port=2
  wires:
  Bus Selector/4 -> MATLAB System/3  "<ydot>"
  Bus Selector/3 -> MATLAB System/2  "<xdot>"
  Bus Selector/5 -> MATLAB System/4  "<ay>"
  Bus Selector/6 -> Sum/2  "<psi>"
  Input/1 -> Bus Selector/1
  Bus Selector/1 -> Matrix Concatenate/1  "<X>"
  Bus Selector/2 -> Matrix Concatenate/2  "<Y>"
  Sum/1 -> PID Controller/1
  PID Controller/1 -> Reshape/1
  Matrix Concatenate/1 -> MATLAB System/1
  Input1/1 -> MATLAB System/5
  MATLAB System/2 -> Sum/1
  MATLAB System/1 -> is_finish/1
  Reshape/1 -> yaw_angle/1

== system VehicleFollowing/Vehicle Model 3 - PID/Subsystem ==
  Input : Inport
  Input1 : Inport  Port=2
  Input2 : Inport  Port=3
  Bus Selector : BusSelector  OutputSignals=InertFrm.Cg.Disp.X,InertFrm.Cg.Disp.Y,InertFrm.Cg.Ang.psi  OutputAsBus=on
  Bus Selector1 : BusSelector  OutputSignals=X,Y,psi
  Bus Selector2 : BusSelector  OutputSignals=InertFrm.Cg.Disp.X,InertFrm.Cg.Disp.Y,InertFrm.Cg.Ang.psi
  MATLAB System : MATLABSystem  System=obstacle_detector  v1_frame=[ 4, 2 ]  v2_frame=[ 4, 2 ]  ego_frame=[ 4, 2 ]  SimulateUsing=Interpreted execution
      mask Type: obstacle_detector
      mask Display:
      | disp('obstacle_detector');
      | port_label('input',1,'v1_pos');
      | port_label('input',2,'v2_X');
      | port_label('input',3,'v2_Y');
      | port_label('input',4,'v2_psi');
      | port_label('input',5,'ego_X');
      | port_label('input',6,'ego_Y');
      | port_label('input',7,'ego_psi');
      | port_label('output',1,'mf_relative_distance');
      | port_label('output',2,'rf_relative_distance');
  MATLAB System1 : MATLABSystem  System=command_generator  SimulateUsing=Interpreted execution
      mask Type: command_generator
      mask Display:
      | disp('command_generator');
      | port_label('input',1,'mf_d');
      | port_label('input',2,'lf_d');
      | port_label('output',1,'command');
  relative_distance : Outport
  Output : Outport  Port=2
  wires:
  MATLAB System/1 -> MATLAB System1/1, relative_distance/1
  Input/1 -> Bus Selector/1
  Bus Selector/1 -> MATLAB System/1
  Input1/1 -> Bus Selector1/1
  Bus Selector1/1 -> MATLAB System/2  "<X>"
  Input2/1 -> Bus Selector2/1
  Bus Selector2/1 -> MATLAB System/5  "<X>"
  Bus Selector2/2 -> MATLAB System/6  "<Y>"
  Bus Selector2/3 -> MATLAB System/7  "<psi>"
  Bus Selector1/2 -> MATLAB System/3  "<Y>"
  Bus Selector1/3 -> MATLAB System/4  "<psi>"
  MATLAB System/2 -> MATLAB System1/2  "rf_rd"
  MATLAB System1/1 -> Output/1

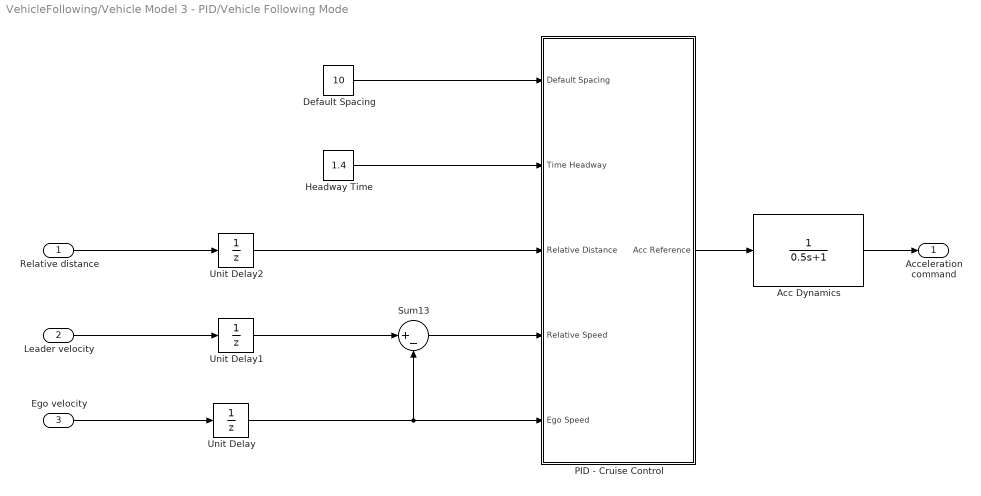
== system VehicleFollowing/Vehicle Model 3 - PID/Vehicle Following Mode ==
  Relative distance : Inport
  Leader velocity : Inport  Port=2
  Ego velocity : Inport  Port=3
  Acc Dynamics : TransferFcn  Denominator=[0.5 1]
  Default Spacing : Constant  Value=10
  Headway Time : Constant  Value=1.4
  PID - Cruise Control : Subsystem
  Sum13 : Sum  Inputs=|+-
  Unit Delay : UnitDelay  SampleTime=-1  HasFrameUpgradeWarning=on
  Unit Delay1 : UnitDelay  SampleTime=-1  HasFrameUpgradeWarning=on
  Unit Delay2 : UnitDelay  SampleTime=-1  HasFrameUpgradeWarning=on
  Acceleration command : Outport
  wires:
  Leader velocity/1 -> Unit Delay1/1
  Headway Time/1 -> PID - Cruise Control/2(Time Headway)
  Ego velocity/1 -> Unit Delay/1
  Sum13/1 -> PID - Cruise Control/4(Relative Speed)
  Relative distance/1 -> Unit Delay2/1
  PID - Cruise Control/1(Acc Reference) -> Acc Dynamics/1
  Acc Dynamics/1 -> Acceleration command/1
  Default Spacing/1 -> PID - Cruise Control/1(Default Spacing)
  Unit Delay/1 -> Sum13/2, PID - Cruise Control/5(Ego Speed)
  Unit Delay1/1 -> Sum13/1
  Unit Delay2/1 -> PID - Cruise Control/3(Relative Distance)

== system VehicleFollowing/Vehicle Model 1 - Manual/Powertrain & Driveline/Brake System ==
  Decc : Inport
  Hydraulics : autolibutils/Cont LPF  wc=30*pi*2  aMode=2
      settings: SourceProductBaseCode=PW,MT,VE,VP
  Pressure : Gain  Gain=2e7
  Saturation1 : Saturate  UpperLimit=inf  LowerLimit=0  ZeroCross=off
  Selector : Selector  InputPortWidth=1  IndexOptions=Index vector (dialog)  Indices=[1 1 1 1]  OutputSizes=1
  Signal Specification : SignalSpecification  Unit=Pa
  Prs : Outport  VectorParamsAs1DForOutWhenUnconnected=off
  wires:
  Pressure/1 -> Selector/1
  Hydraulics/1 -> Pressure/1
  Saturation1/1 -> Hydraulics/1
  Selector/1 -> Signal Specification/1
  Decc/1 -> Saturation1/1
  Signal Specification/1 -> Prs/1
